simulink model "Week3_Problem1"  (R2020b)
settings: Solver=FixedStepDiscrete  StartTime=0.0  StopTime=200  FixedStep=0.1  MaxStep=0.1  RelTol=1e-3  EnableMultiTasking=on
undefined symbols (not defined in the file): sigbuilder_block
settings Model: Creator=hp  LastModifiedBy=hp
settings DataIOCC: SaveFormat=Array  ReturnWorkspaceOutputs=off

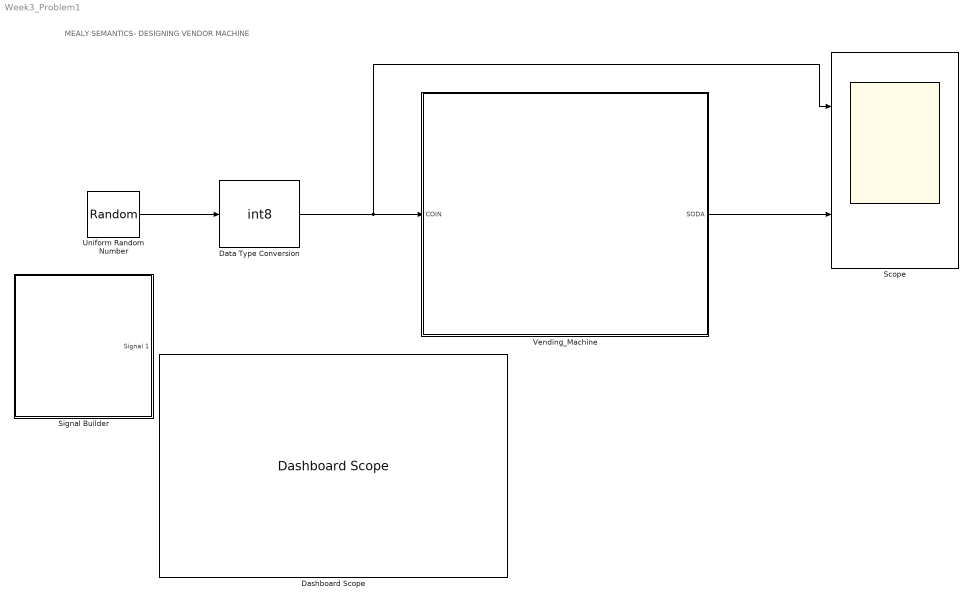
== system Week3_Problem1 ==
  note: MEALY SEMANTICS- DESIGNING VENDOR MACHINE
  Dashboard Scope : DashboardScope
  Data Type Conversion : DataTypeConversion  OutDataTypeStr=int8  RndMeth=Nearest  SaturateOnIntegerOverflow=on
  Scope : Scope  NumInputPorts=2
  Signal Builder : Subsystem  Tag=STV Subsys  LoadFcn=sigbuilder_block('load');  StartFcn=sigbuilder_block('start');  StopFcn=sigbuilder_block('stop');  ClipboardFcn=sigbuilder_block('clipboard');  mask(Sigbuilder block){tuvar=[0:10]}
      mask help: Simulink:masks:SigbuilderBlock_MD
      mask init:
      | if ~strcmp(get_param(bdroot(gcbh),'SimulationStatus'),'stopped') tuvar = sigbuilder_block('maskInit'); end
      settings: CopyFcn=sigbuilder_block('copy');  DeleteFcn=sigbuilder_block('delete');  ModelCloseFcn=sigbuilder_block('modelClose');  PreSaveFcn=sigbuilder_block('preSave');  PauseFcn=sigbuilder_block('pause');  ContinueFcn=sigbuilder_block('continue');  NameChangeFcn=sigbuilder_block('namechange');  OpenFcn=sigbuilder_block('open',[444.75 12 550.5 359.25 ]);  CloseFcn=sigbuilder_block('close');
      mask Display: plot(0, 0, 100, 100,[2, 2, 32, 32, 2], [68, 8, 8, 68, 68],[32, 2], [38, 38], [32, 19, 2],[53, 60, 44], [32, 17, 17, 2],[16, 16, 31, 31]);txt = getActiveGroup(gcbh);text(2, 100, txt,'verticalAlignment', 'top');
  Uniform Random Number : UniformRandomNumber  Minimum=0  Maximum=2  Seed=337  SampleTime=10
  Vending_Machine : Stateflow chart  TreatAsAtomicUnit=on
  wires:
  Vending_Machine/1(SODA) -> Scope/2
  Data Type Conversion/1 -> Vending_Machine/1(COIN), Scope/1
  Uniform Random Number/1 -> Data Type Conversion/1

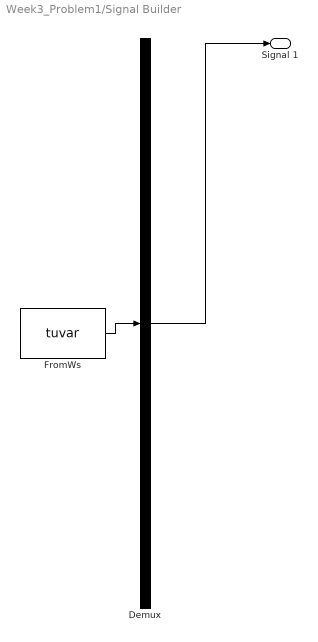
== system Week3_Problem1/Signal Builder ==
  Demux : Demux  Tag=STV Demux  Outputs=1
      settings: DisplayOption=none
  FromWs : FromWorkspace  Tag=STV FromWs  VariableName=tuvar
      SigBuilderData=|
      | common.afterFinalStr = 'Extrapolate'
      | common.sampleTime = 0
      | dataSet.timeRange = [0 200]
      | dataSet.name = 'Group 1'
      | sbobj.Groups.Name = 'Group 1'
      | sbobj.Groups.Signals.Name = 'Signal 1'
      | sbobj.Groups.Signals.XData = [0 4 4 6 6 68.5 68.5 99.5 99.5 140 140 170 170 188 188 200]
      | sbobj.Groups.Signals.YData = [2 2 1 1 0 0 1 1 2 2 1 1 2 2 1 1]
      | sbobj.Groups.TimeRange = [0 200]
  Signal 1 : Outport  Tag=STV Outport
  wires:
  Demux/1 -> Signal 1/1
  FromWs/1 -> Demux/1

== stateflow chart Week3_Problem1/Vending_Machine ==
  settings: stateMachineType=MEALY_MACHINE  initializeOutput=1
  state INITIAL_STATE
  state NICKEL_STATE
  state DIME_STATE
  (default) -> INITIAL_STATE
  INITIAL_STATE -> NICKEL_STATE [order 1] : [COIN==1]{SODA=0}
  NICKEL_STATE -> INITIAL_STATE [order 2] : [COIN==2]{SODA=1}
  DIME_STATE -> INITIAL_STATE [order 1] : [COIN==1]{SODA=1}
  INITIAL_STATE -> DIME_STATE [order 2] : [COIN==2]{SODA=0}
  NICKEL_STATE -> DIME_STATE [order 1] : [COIN==1]{SODA=0}
  DIME_STATE -> NICKEL_STATE [order 2] : [COIN==2]{SODA=1}
  data: COIN input; SODA output double
